simulink model "runSfunWithCoeffsOnly"  (R2019b)
settings: Solver=FixedStepDiscrete  StartTime=tstart  StopTime=tend  FixedStep=Ts  RelTol=1e-3  EnableMultiTasking=on
settings Model: PauseTimes=341.0  Creator=btc2abt  LastModifiedBy=IGG2BP
settings DataIOCC: LimitDataPoints=on  ReturnWorkspaceOutputs=off
settings OptimizationCC: LifeSpan=inf
settings DebuggingCC: MultiTaskRateTransMsg=warning  AllowSymbolicDim=off  SFUnexpectedBacktrackingDiag=warning  SFNoUnconditionalDefaultTransitionDiag=warning  SFExecutionAtInitializationDiag=none  ArithmeticOperatorsInVariantConditions=warning
settings ModelReferenceCC: PropagateSignalLabelsOutOfModel=off
settings SFSimCC: SimUseLocalCustomCode=off  CustomCodeUndefinedFunction=UseInterfaceOnly
settings RTWCC: RTWUseLocalCustomCode=off
settings CodeAppCC: StateflowObjectComments=on
settings GRTTargetCC: TargetLangStandard=C89/C90 (ANSI)
settings ConfigComp: CovMetricSettings=dw  CovHtmlReporting=on  CovSaveCumulativeToWorkspaceVar=on  CovSaveSingleToWorkspaceVar=on  CovExternalEMLEnable=off

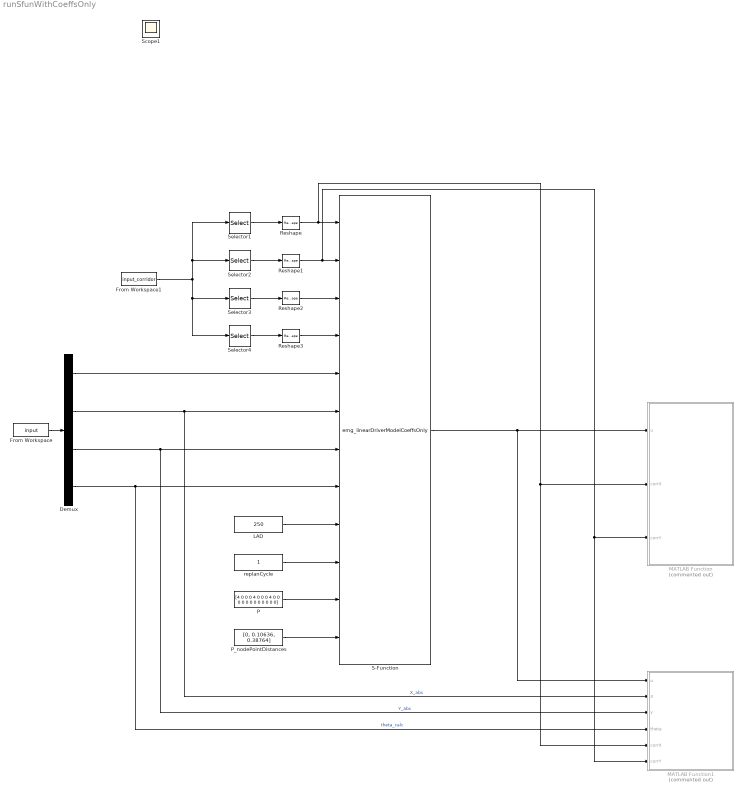
== system runSfunWithCoeffsOnly ==
  Demux : Demux
  From Workspace : FromWorkspace  VariableName=input  SampleTime=0  Interpolate=off  OutputAfterFinalValue=Holding final value
  From Workspace1 : FromWorkspace  VariableName=input_corridor  SampleTime=0  Interpolate=off  OutputAfterFinalValue=Holding final value
  LAD : Constant  Value=250
  MATLAB Function : MATLAB Function  Commented=on  TreatAsAtomicUnit=on
  MATLAB Function1 : MATLAB Function  Commented=on  TreatAsAtomicUnit=on
  P : Constant  Value=[4 0 0 0 4 0 0 0 4 0 0 0 0 0 0 0 0 0 0 0 0]
  P_nodePointDistances : Constant  Value=[0, 0.10636, 0.38764]
  Reshape{,1..3} (4 alike) : Reshape
  S-Function : S-Function  FunctionName=emg_linearDriverModelCoeffsOnly  SFunctionDeploymentMode=off  EnableBusSupport=off
  Selector1 : Selector  NumberOfDimensions=2  InputPortWidth=3  IndexOptions=Index vector (dialog),Select all  Indices=[1],1  OutputSizes=1,1
  Selector2 : Selector  NumberOfDimensions=2  InputPortWidth=3  IndexOptions=Index vector (dialog),Select all  Indices=[2],1  OutputSizes=1,1
  Selector3 : Selector  NumberOfDimensions=2  InputPortWidth=3  IndexOptions=Index vector (dialog),Select all  Indices=[3],1  OutputSizes=1,1
  Selector4 : Selector  NumberOfDimensions=2  InputPortWidth=3  IndexOptions=Index vector (dialog),Select all  Indices=[4],1  OutputSizes=1,1
  replanCycle : Constant
  Scope1 : Scope
  wires:
  P/1 -> S-Function/11
  P_nodePointDistances/1 -> S-Function/12
  replanCycle/1 -> S-Function/10
  LAD/1 -> S-Function/9
  From Workspace/1 -> Demux/1
  From Workspace1/1 -> Selector1/1, Selector2/1, Selector3/1, Selector4/1
  Selector1/1 -> Reshape/1
  Selector2/1 -> Reshape1/1
  Selector3/1 -> Reshape2/1
  Selector4/1 -> Reshape3/1
  S-Function/1 -> MATLAB Function1/1(u), MATLAB Function/1(u)
  Demux/1 -> S-Function/5
  Demux/2 -> MATLAB Function1/2(X), S-Function/6  "X_abs"
  Demux/3 -> MATLAB Function1/3(Y), S-Function/7  "Y_abs"
  Demux/4 -> MATLAB Function1/4(theta), S-Function/8  "theta_calc"
  Reshape/1 -> MATLAB Function1/5(corrX), MATLAB Function/2(corrX), S-Function/1
  Reshape1/1 -> MATLAB Function1/6(corrY), MATLAB Function/3(corrY), S-Function/2
  Reshape2/1 -> S-Function/3
  Reshape3/1 -> S-Function/4

== matlab function runSfunWithCoeffsOnly/MATLAB Function1 ==
  data: u input; X input; Y input; theta input; corrX input; corrY input
function fcn(u, X,Y,theta, corrX, corrY)
% creating the global trajectory point
if (~all(u==0))
    trajGlobalX = X - sin(theta)*u(1);
    trajGlobalY = Y + cos(theta)*u(1);
    
    corGlobalX = X - sin(theta)*corrY(1);
    corGlobalY = Y + cos(theta)*corrY(1);
    
    corLeftX = X - sin(theta)*(1.875);
    corLeftY = Y + cos(theta)*(1.875);

    plot(trajGlobalX, trajGlobalY, 'bo', corGlobalX, corGlobalY, 'k*', corLeftX, corLeftY, 'kx');
    grid on;
    hold on;
    plot(X,Y,'rx');
    pause(0.1);
    xlim([X-5, X+5]); ylim([Y-5, Y+5]);
end

== matlab function runSfunWithCoeffsOnly/MATLAB Function ==
  data: u input; corrX input; corrY input
function fcn(u, corrX, corrY)
if (~all(u==0))
    x = linspace(0,u(5), 100);
    y = u(1)+u(2)*x+u(3)/2*x.^2+u(4)/6*x.^3;
    plot(corrX, corrY, 'bo', x,y, 'rx');
    %legend('cor', 'traj');
    grid on;
    xlim([0,150]);
    ylim([-5,5]);
    pause(0.1);
    %axis equal;
end
